simulink model "schema_deadbeat_testare_num"  (R2023a)
settings: Solver=VariableStepAuto  StartTime=0.0  StopTime=20  RelTol=1e-3
values from neighbouring files (symbols this model uses):
  Ts2 = 0.4    [Untitled.m]
undefined symbols (not defined in the file or in its folder): den0_dead, denp_dead, denrs_dead, num0_dead, nump_dead, numrs_dead
settings Model: LastModifiedBy=Traxar72
settings RTWCC: GPUComputeCapability=5.0

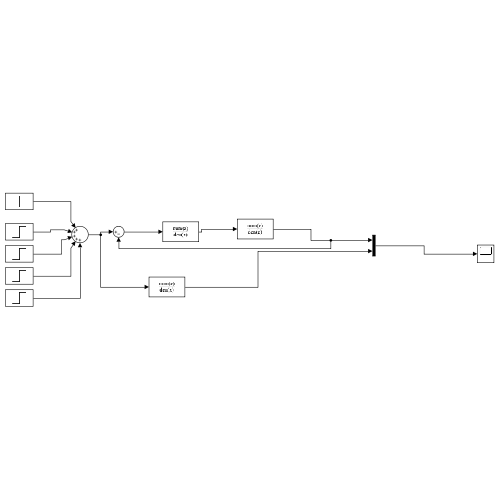
[thumbnail: Simulink's stored preview of the top-level diagram]
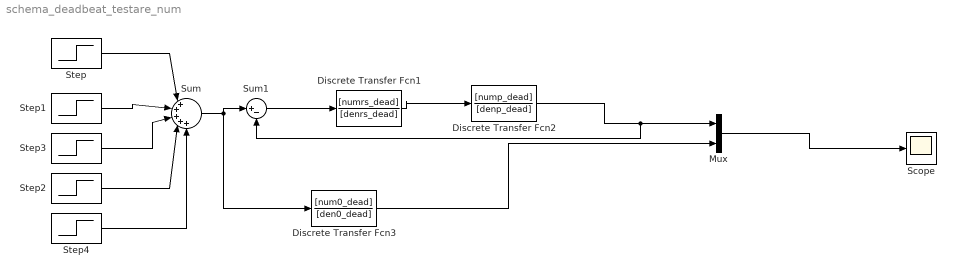
== system schema_deadbeat_testare_num ==
  Discrete Transfer Fcn1 : DiscreteTransferFcn  Numerator=[numrs_dead]  Denominator=[denrs_dead]  SampleTime=Ts2
  Discrete Transfer Fcn2 : DiscreteTransferFcn  Numerator=[nump_dead]  Denominator=[denp_dead]  SampleTime=Ts2
  Discrete Transfer Fcn3 : DiscreteTransferFcn  Numerator=[num0_dead]  Denominator=[den0_dead]  SampleTime=Ts2
  Mux : Mux  Inputs=2
  Scope : Scope
  Step : Step  Time=16  After=-4  SampleTime=Ts2
  Step1 : Step  Time=12  SampleTime=Ts2
  Step2 : Step  Time=4  SampleTime=Ts2
  Step3 : Step  Time=8  SampleTime=Ts2
  Step4 : Step  Time=0  SampleTime=Ts2
  Sum : Sum  Inputs=|+++++
  Sum1 : Sum  Inputs=|+-
  wires:
  Step/1 -> Sum/1
  Step1/1 -> Sum/2
  Step3/1 -> Sum/3
  Step2/1 -> Sum/4
  Step4/1 -> Sum/5
  Sum/1 -> Discrete Transfer Fcn3/1, Sum1/1
  Discrete Transfer Fcn1/1 -> Discrete Transfer Fcn2/1
  Discrete Transfer Fcn3/1 -> Mux/2
  Mux/1 -> Scope/1
  Sum1/1 -> Discrete Transfer Fcn1/1
  Discrete Transfer Fcn2/1 -> Sum1/2, Mux/1
